simulink library "calculateCYorCLorCN_ul"  (R2020a)
settings: Solver=VariableStepAuto  StartTime=0.0  StopTime=10.0  RelTol=1e-3
undefined symbols (not defined in the file or in its folder): coeffvals
libraries: calcAeroCoeffFromPolynomial_ul x5
settings Model: Creator=Ayaz  LastModifiedBy=Ayaz

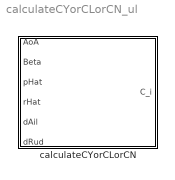
== system calculateCYorCLorCN_ul ==
  calculateCYorCLorCN : Subsystem  mask{C_i_Beta_coeffs=coeffvals, C_i_pHat_coeffs=coeffvals, C_i_rHat_coeffs=coeffvals, C_i_dAil_coeffs=coeffvals, C_i_dRud_coeffs=coeffvals}
      mask prompts: C_i_Beta_coeffs "C_i_Beta polynomial coefficients (c0,c1,c2):"; C_i_pHat_coeffs "C_i_pHat polynomial coefficients (c0,c1,c2):"; C_i_rHat_coeffs "C_i_rHat polynomial coefficients (c0,c1,c2):"; C_i_dAil_coeffs "C_i_dAil polynomial coefficients (c0,c1,c2):"; C_i_dRud_coeffs "C_i_dRud polynomial coefficients (c0,c1,c2):"
      mask TypeOptions C_i_Beta_coeffs: C_i_Beta/coeffVals
      mask TypeOptions C_i_pHat_coeffs: C_i_pHat/coeffVals
      mask TypeOptions C_i_rHat_coeffs: C_i_rHat/coeffVals
      mask TypeOptions C_i_dAil_coeffs: C_i_dAil/coeffVals
      mask TypeOptions C_i_dRud_coeffs: C_i_dRud/coeffVals

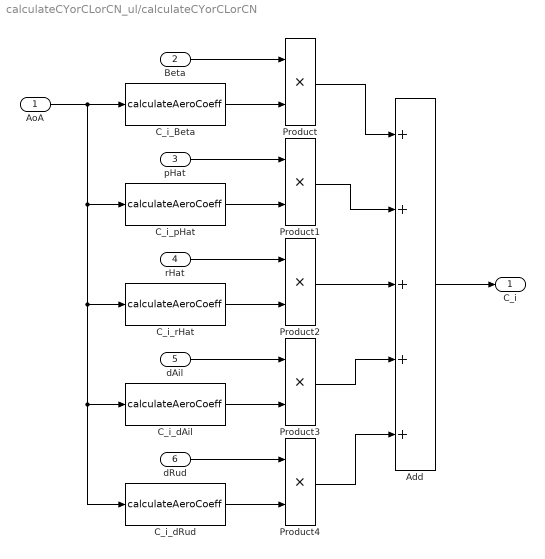
== system calculateCYorCLorCN_ul/calculateCYorCLorCN ==
  AoA : Inport
  Beta : Inport  Port=2
  pHat : Inport  Port=3
  rHat : Inport  Port=4
  dAil : Inport  Port=5
  dRud : Inport  Port=6
  Add : Sum  Inputs=+++++
  C_i_Beta : calcAeroCoeffFromPolynomial_ul/calculateAeroCoeff  coeffVals=C_i_Beta_coeffs
  C_i_dAil : calcAeroCoeffFromPolynomial_ul/calculateAeroCoeff  coeffVals=C_i_dAil_coeffs
  C_i_dRud : calcAeroCoeffFromPolynomial_ul/calculateAeroCoeff  coeffVals=C_i_dRud_coeffs
  C_i_pHat : calcAeroCoeffFromPolynomial_ul/calculateAeroCoeff  coeffVals=C_i_pHat_coeffs
  C_i_rHat : calcAeroCoeffFromPolynomial_ul/calculateAeroCoeff  coeffVals=C_i_rHat_coeffs
  Product{,1..4} (5 alike) : Product
  C_i : Outport
  wires:
  Beta/1 -> Product/1
  pHat/1 -> Product1/1
  rHat/1 -> Product2/1
  dAil/1 -> Product3/1
  dRud/1 -> Product4/1
  Add/1 -> C_i/1
  AoA/1 -> C_i_dRud/1, C_i_dAil/1, C_i_rHat/1, C_i_pHat/1, C_i_Beta/1
  C_i_Beta/1 -> Product/2
  C_i_pHat/1 -> Product1/2
  C_i_rHat/1 -> Product2/2
  C_i_dAil/1 -> Product3/2
  C_i_dRud/1 -> Product4/2
  Product/1 -> Add/1
  Product1/1 -> Add/2
  Product2/1 -> Add/3
  Product3/1 -> Add/4
  Product4/1 -> Add/5
